simulink model "Xcvr_SSB_AM_2p5"  (Simulink 7.4)
settings: Solver=VariableStepDiscrete  SolverMode=SingleTasking  StartTime=0.0  StopTime=10  RelTol=1e-3
PreLoadFcn:
  | Fs=80e6;
  | 
  | phee=da_rom();
  | [phee_1,phee_2]=da_i2_rom();
  | 
  | Dcic=64;       % CIC decimation
  | Dfac=128;    % following DA filter decimation
  | N = 6;           %       (2^(N+1))=Dfac
  | Daudio=Dcic*Dfac;
  | Faudio=Fs/Daudio;
  | 
  | load info_filt_ssb_4
  | load Serial_Intfc_Stream_5
  | 
  | % AGC related
  | x=0.5:1/256:(1-1/256);
  | addr=(x-0.5)*256;
  | y=1./x;
undefined symbols (not defined in the file): Serial_Interface, ssb_coef, xlipgetpartsetting
libraries: xbsIndex_r4 x1305, dspsrcs4 x5, simulink x2, dspsigops x2, dspsnks4 x1
(part 2 of 11)

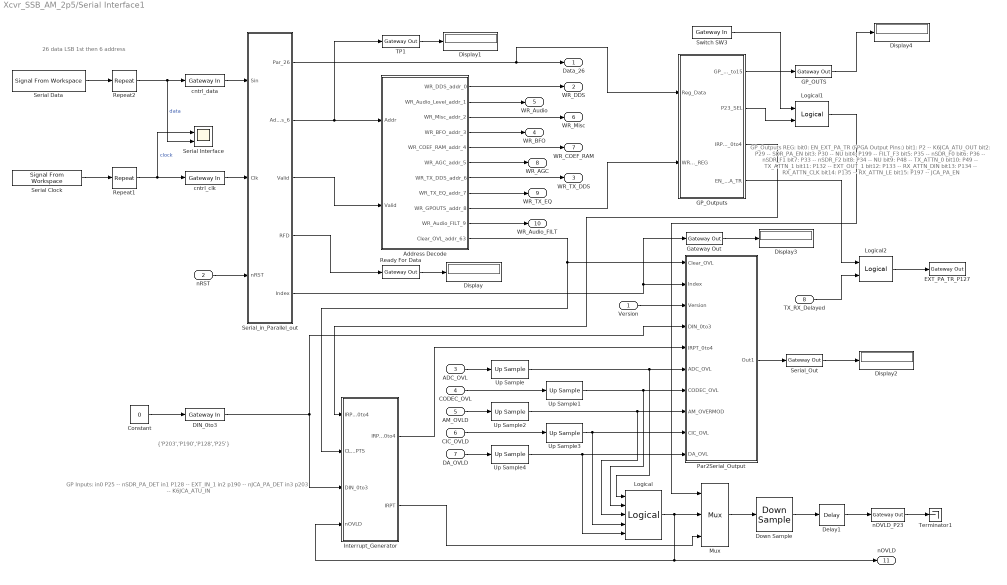
== system Xcvr_SSB_AM_2p5/Serial Interface1 ==
  note: 26 data  LSB 1st
      | then 6 address
  note: {'P203','P190','P128','P25'}
  note: GP Inputs:
      | in0  P25 -- nSDR_PA_DET
      | in1  P128 -- EXT_IN_1
      | in2  p190 -- nJCA_PA_DET
      | in3  p203 -- K6JCA_ATU_IN
  note: GP_Outputs REG:
      |
      | bit0: EN_EXT_PA_TR
      |
      | (FPGA Output Pins:)
      | bit1: P2 -- K6JCA_ATU_OUT
      | bit2: P29 -- SDR_PA_EN
      | bit3: P30 -- NU
      | bit4: P199 -- FILT_F3
      | bit5: P35 --  nSDR_F0
      | bit6: P36 -- nSDR_F1
      | bit7: P33 -- nSDR_F2
      | bit8: P34 -- NU
      |
      | bit9: P48 -- TX_ATTN_0
      | bit10: P49 -- TX_ATTN_1
      | bit11: P132 -- EXT_OUT_1
      | bit12: P133 -- RX_ATTN_DIN
      | bit13: P134 -- RX_ATTN_CLK
      | bit14: P135 -- RX_ATTN_LE
      | bit15: P197 -- JCA_PA_EN
  Version : Inport  OutDataType=fixdt(1, 16)  OutScaling=2^0
  nRST : Inport  Port=2  OutDataType=fixdt(1, 16)  OutScaling=2^0
  ADC_OVL : Inport  Port=3  OutDataType=fixdt(1, 16)  OutScaling=2^0
  CODEC_OVL : Inport  Port=4  OutDataType=fixdt(1, 16)  OutScaling=2^0
  AM_OVLD : Inport  Port=5  OutDataType=fixdt(1, 16)  OutScaling=2^0
  CIC_OVLD : Inport  Port=6  OutDataType=fixdt(1, 16)  OutScaling=2^0
  DA_OVLD : Inport  Port=7  OutDataType=fixdt(1, 16)  OutScaling=2^0
  TX_RX_Delayed : Inport  Port=8  OutDataType=fixdt(1, 16)  OutScaling=2^0
  Address Decode : Subsystem
  Constant : Constant  Value=0  OutDataType=fixdt(1, 16)  OutScaling=2^0  SampleTime=8/Fs
  DIN_0to3 : xbsIndex_r4/Gateway In  arith_type=Unsigned  n_bits=4  bin_pt=0  quantization="Round  (unbiased: +/- Inf)"  overflow=Wrap  period=8/Fs  dbl_ovrd=off  timing_constraint=None  locs_specified=on  LOCs={'P203','P190','P128','P25'}  hdl_port=on  block_type=gatewayin
      settings: infoedit="Gateway in block.  Converts inputs of type Simulink integer, double and fixed point to  Xilinx fixed point type.<br><br>Hardware notes:  In hardware these blocks become top level input ports."  block_version=9.2.00
  Delay1 : xbsIndex_r4/Delay  en=off  latency=1  dbl_ovrd=off  reg_retiming=off  block_type=delay
      settings: block_version=12.1
  Display{,1..4} (5 alike) : Display
  Down Sample : xbsIndex_r4/Down Sample  sample_ratio=1024  sample_phase="Last Value of Frame  (most efficient)"  en=off  latency=1  dbl_ovrd=off  block_type=dsamp
      settings: block_version=12.1
  EXT_PA_TR_P127 : xbsIndex_r4/Gateway Out  hdl_port=on  timing_constraint=None  locs_specified=on  LOCs={'P127'}  block_type=gatewayout
      settings: infoedit="Gateway out block.  Converts Xilinx fixed point inputs into ouputs of type Simulink integer, double, or fixed point.<br><br>Hardware notes:  In hardware these blocks become top level output ports or are discarded, depending on how they are configured."  block_version=12.1
  GP_OUTS : xbsIndex_r4/Gateway Out  hdl_port=on  timing_constraint=None  locs_specified=on  LOCs={'P197','P135','P134','P133','P132','P49','P48','P34','P33','P36','P35','P199','P30','P29','P2'}  block_type=gatewayout
      settings: infoedit="Gateway out block.  Converts Xilinx fixed point inputs into ouputs of type Simulink integer, double, or fixed point.<br><br>Hardware notes:  In hardware these blocks become top level output ports or are discarded, depending on how they are configured."  block_version=12.1
  GP_Outputs : Subsystem
  Gateway Out : xbsIndex_r4/Gateway Out  hdl_port=off  timing_constraint=None  locs_specified=off  LOCs={}  block_type=gatewayout
      settings: infoedit="Gateway out block.  Converts Xilinx fixed point inputs into ouputs of type Simulink integer, double, or fixed point.<br><br>Hardware notes:  In hardware these blocks become top level output ports or are discarded, depending on how they are configured."  block_version=12.1
  Interrupt_Generator : Subsystem
  Logical : xbsIndex_r4/Logical  logical_function=NOR  inputs=5  en=off  latency=0  precision=Full  arith_type=Unsigned  n_bits=16  bin_pt=0  align_bp=on  dbl_ovrd=off  block_type=logical
      settings: block_version=12.1
  Logical1 : xbsIndex_r4/Logical  logical_function=OR  inputs=2  en=off  latency=0  precision=Full  arith_type=Unsigned  n_bits=16  bin_pt=0  align_bp=on  dbl_ovrd=off  block_type=logical
      settings: block_version=12.1
  Logical2 : xbsIndex_r4/Logical  logical_function=AND  inputs=2  en=off  latency=0  precision=Full  arith_type=Unsigned  n_bits=16  bin_pt=0  align_bp=on  dbl_ovrd=off  block_type=logical
      settings: block_version=12.1
  Mux : xbsIndex_r4/Mux  inputs=2  en=off  latency=0  precision=Full  arith_type=Unsigned  n_bits=16  bin_pt=14  quantization=Truncate  overflow=Wrap  dbl_ovrd=off  block_type=mux
      settings: block_version=12.1
  Par2Serial_Output : Subsystem
  Ready For Data : xbsIndex_r4/Gateway Out  hdl_port=on  timing_constraint=None  locs_specified=on  LOCs={'P18'}  block_type=gatewayout
      settings: infoedit="Gateway out block.  Converts Xilinx fixed point inputs into ouputs of type Simulink integer, double, or fixed point.<br><br>Hardware notes:  In hardware these blocks become top level output ports or are discarded, depending on how they are configured."  block_version=12.1
  Repeat1 : dspsigops/Repeat  N=3*6  ic=0  mode=Maintain input frame size
  Repeat2 : dspsigops/Repeat  N=3*6  ic=0  mode=Maintain input frame size
  "Serial Clock  " : dspsrcs4/Signal From Workspace  SystemSampleTime=-1  X=Serial_Interface(1,:)  Ts=3*48/Fs  nsamps=1  OutputAfterFinalValue=Holding final value  ignoreOrWarnInputAndFrameLengths=off
  Serial Data : dspsrcs4/Signal From Workspace  SystemSampleTime=-1  X=Serial_Interface(2,:)  Ts=3*48/Fs  nsamps=1  OutputAfterFinalValue=Holding final value  ignoreOrWarnInputAndFrameLengths=off
  Serial Interface : Scope  NumInputPorts=2
      settings: YMin=-5~-5  YMax=5~5  SaveName=ScopeData3
  Serial_Out : xbsIndex_r4/Gateway Out  hdl_port=on  timing_constraint=None  locs_specified=on  LOCs={'P19'}  block_type=gatewayout
      settings: infoedit="Gateway out block.  Converts Xilinx fixed point inputs into ouputs of type Simulink integer, double, or fixed point.<br><br>Hardware notes:  In hardware these blocks become top level output ports or are discarded, depending on how they are configured."  block_version=12.1
  Serial_in_Parallel_out : Subsystem
  Switch SW3 : xbsIndex_r4/Gateway In  arith_type=Boolean  n_bits=1  bin_pt=0  quantization="Round  (unbiased: +/- Inf)"  overflow=Saturate  period=1/Faudio  dbl_ovrd=off  timing_constraint=None  locs_specified=on  LOCs={'P90'}  hdl_port=on  block_type=gatewayin
      settings: infoedit="Gateway in block.  Converts inputs of type Simulink integer, double and fixed point to  Xilinx fixed point type.<br><br>Hardware notes:  In hardware these blocks become top level input ports."  block_version=9.2.00
  TP1 : xbsIndex_r4/Gateway Out  hdl_port=off  timing_constraint=None  locs_specified=off  LOCs={'P11'}  block_type=gatewayout
      settings: infoedit="Gateway out block.  Converts Xilinx fixed point inputs into ouputs of type Simulink integer, double, or fixed point.<br><br>Hardware notes:  In hardware these blocks become top level output ports or are discarded, depending on how they are configured."  block_version=12.1
  Terminator1 : Terminator
  Up Sample : xbsIndex_r4/Up Sample  sample_ratio=8  copy_samples=on  en=off  latency=0  dbl_ovrd=off  block_type=usamp
      settings: block_version=12.1
  Up Sample1 : xbsIndex_r4/Up Sample  sample_ratio=1024  copy_samples=on  en=off  latency=0  dbl_ovrd=off  block_type=usamp
      settings: block_version=12.1
  Up Sample2 : xbsIndex_r4/Up Sample  sample_ratio=1024  copy_samples=on  en=off  latency=0  dbl_ovrd=off  block_type=usamp
      settings: block_version=12.1
  Up Sample3 : xbsIndex_r4/Up Sample  sample_ratio=8  copy_samples=on  en=off  latency=0  dbl_ovrd=off  block_type=usamp
      settings: block_version=12.1
  Up Sample4 : xbsIndex_r4/Up Sample  sample_ratio=8  copy_samples=on  en=off  latency=0  dbl_ovrd=off  block_type=usamp
      settings: block_version=12.1
  cntrl_clk : xbsIndex_r4/Gateway In  arith_type=Boolean  n_bits=16  bin_pt=14  quantization="Round  (unbiased: +/- Inf)"  overflow=Saturate  period=8/Fs  dbl_ovrd=off  timing_constraint=None  locs_specified=on  LOCs={'P16'}  hdl_port=on  block_type=gatewayin
      settings: infoedit="Gateway in block.  Converts inputs of type Simulink integer, double and fixed point to  Xilinx fixed point type.<br><br>Hardware notes:  In hardware these blocks become top level input ports."  block_version=9.2.00
  cntrl_data : xbsIndex_r4/Gateway In  arith_type=Boolean  n_bits=16  bin_pt=14  quantization="Round  (unbiased: +/- Inf)"  overflow=Saturate  period=8/Fs  dbl_ovrd=off  timing_constraint=None  locs_specified=on  LOCs={'P15'}  hdl_port=on  block_type=gatewayin
      settings: infoedit="Gateway in block.  Converts inputs of type Simulink integer, double and fixed point to  Xilinx fixed point type.<br><br>Hardware notes:  In hardware these blocks become top level input ports."  block_version=9.2.00
  nOVLD_P23 : xbsIndex_r4/Gateway Out  hdl_port=on  timing_constraint=None  locs_specified=on  LOCs={'P23'}  block_type=gatewayout
      settings: infoedit="Gateway out block.  Converts Xilinx fixed point inputs into ouputs of type Simulink integer, double, or fixed point.<br><br>Hardware notes:  In hardware these blocks become top level output ports or are discarded, depending on how they are configured."  block_version=9.2.00
  Data_26 : Outport
  WR_DDS : Outport  Port=2
  WR_TX_DDS : Outport  Port=3
  WR_BFO : Outport  Port=4
  WR_Audio : Outport  Port=5
  WR_Misc : Outport  Port=6
  WR_COEF_RAM : Outport  Port=7
  WR_AGC : Outport  Port=8
  WR_TX_EQ : Outport  Port=9
  WR_Audio_FILT : Outport  Port=10
  nOVLD : Outport  Port=11
  wires:
  cntrl_data/1 -> Serial_in_Parallel_out/1(Sin)
  cntrl_clk/1 -> Serial_in_Parallel_out/2(Clk)
  Serial_in_Parallel_out/2(Address_6) -> Address Decode/1(Addr), TP1/1
  Serial_in_Parallel_out/3(Valid) -> Address Decode/2(Valid)
  Address Decode/2(WR_Audio_Level_addr_1) -> WR_Audio/1
  Serial_in_Parallel_out/1(Par_26) -> Data_26/1, GP_Outputs/1(Reg_Data)
  Address Decode/1(WR_DDS_addr_0) -> WR_DDS/1
  Address Decode/4(WR_BFO_addr_3) -> WR_BFO/1
  Address Decode/3(WR_Misc_addr_2) -> WR_Misc/1
  Address Decode/5(WR_COEF_RAM_addr_4) -> WR_COEF_RAM/1
  Repeat2/1 -> Serial Interface/2, cntrl_data/1  "data"
  Serial Data/1 -> Repeat2/1
  "Serial Clock  "/1 -> Repeat1/1
  Repeat1/1 -> Serial Interface/1, cntrl_clk/1  "clock"
  Ready For Data/1 -> Display/1
  Serial_in_Parallel_out/4(RFD) -> Ready For Data/1
  TP1/1 -> Display1/1
  Serial_in_Parallel_out/5(Index) -> Par2Serial_Output/2(Index), Gateway Out/1
  DIN_0to3/1 -> Par2Serial_Output/4(DIN_0to3), Interrupt_Generator/3(DIN_0to3)
  Version/1 -> Par2Serial_Output/3(Version)
  Par2Serial_Output/1(Out1) -> Serial_Out/1
  Serial_Out/1 -> Display2/1
  Constant/1 -> DIN_0to3/1
  ADC_OVL/1 -> Up Sample/1
  CODEC_OVL/1 -> Up Sample1/1
  Gateway Out/1 -> Display3/1
  Up Sample/1 -> Par2Serial_Output/6(ADC_OVL), Logical/1
  Up Sample1/1 -> Par2Serial_Output/7(CODEC_OVL), Logical/2
  Up Sample2/1 -> Par2Serial_Output/8(AM_OVERMOD), Logical/3
  AM_OVLD/1 -> Up Sample2/1
  Up Sample3/1 -> Par2Serial_Output/9(CIC_OVL), Logical/4
  CIC_OVLD/1 -> Up Sample3/1
  Up Sample4/1 -> Par2Serial_Output/10(DA_OVL), Logical/5
  DA_OVLD/1 -> Up Sample4/1
  Address Decode/6(WR_AGC_addr_5) -> WR_AGC/1
  Address Decode/7(WR_TX_DDS_addr_6) -> WR_TX_DDS/1
  nRST/1 -> Serial_in_Parallel_out/3(nRST)
  nOVLD_P23/1 -> Terminator1/1
  Delay1/1 -> nOVLD_P23/1
  Logical/1 -> Mux/2, Interrupt_Generator/4(nOVLD), nOVLD/1
  Interrupt_Generator/2(IRPT) -> Mux/3
  Interrupt_Generator/1(IRPT_0to4) -> Par2Serial_Output/5(IRPT_0to4)
  GP_Outputs/2(P23_SEL) -> Logical1/2
  Switch SW3/1 -> Logical1/1
  Logical1/1 -> Mux/1
  GP_Outputs/1(GP_OUT_BIT_1_to15) -> GP_OUTS/1
  GP_OUTS/1 -> Display4/1
  Mux/1 -> Down Sample/1
  Down Sample/1 -> Delay1/1
  GP_Outputs/3(IRPT_EN_0to4) -> Interrupt_Generator/1(IRPT_EN_0to4)
  Address Decode/8(WR_TX_EQ_addr_7) -> WR_TX_EQ/1
  Address Decode/9(WR_GPOUTS_addr_8) -> GP_Outputs/2(WR_GP_REG)
  Address Decode/11(Clear_OVL_addr_63) -> Par2Serial_Output/1(Clear_OVL), Interrupt_Generator/2(CLR_IRPTS)
  Address Decode/10(WR_Audio_FILT_9) -> WR_Audio_FILT/1
  Logical2/1 -> EXT_PA_TR_P127/1
  GP_Outputs/4(EN_EXT_PA_TR) -> Logical2/1
  TX_RX_Delayed/1 -> Logical2/2

== system Xcvr_SSB_AM_2p5/TX Filters I=8192 ==
  Real_In : Inport
  Imag_In : Inport  Port=2
  " Sample Rate" : Display
  " Sample Rate1" : Display
  "CIC Compiler 2.0 " : xbsIndex_r4/CIC Compiler 2.0   filter_type=Interpolation  number_of_stages=5  differential_delay=1  number_of_channels=1  sample_rate_changes=Fixed  fixed_or_initial_rate=64  minimum_rate=4  maximum_rate=4  ratespecification=Hardware_Oversampling_Rate  sampleperiod=4  hardwareoversamplingrate=1  quantization=Truncation  output_data_width=16  use_xtreme_dsp_slice=on  use_streaming_interface=on  sclr=off  ce=off  gui_behaviour=Sysgen  input_data_width=18  ip_name=CIC Compiler  ip_version=2.0  dsptool_ready=true  wrapper_available=true  port_translation_map={ 'ce' => 'en', 'sclr' => 'rst' }  ipcore_xco_need_fpga_part=true  ipcore_fpga_part=xlipgetpartsetting(gcb, {'virtex4', 'xc4vsx35', '-10', 'ff668'})  ipcore_verbose=false  block_type=cic_compiler_v2_0
      settings: block_version=12.1
  CIC Compiler 2.0 1 : xbsIndex_r4/CIC Compiler 2.0   filter_type=Interpolation  number_of_stages=5  differential_delay=1  number_of_channels=1  sample_rate_changes=Fixed  fixed_or_initial_rate=64  minimum_rate=4  maximum_rate=4  ratespecification=Hardware_Oversampling_Rate  sampleperiod=4  hardwareoversamplingrate=1  quantization=Truncation  output_data_width=16  use_xtreme_dsp_slice=on  use_streaming_interface=on  sclr=off  ce=off  gui_behaviour=Sysgen  input_data_width=18  ip_name=CIC Compiler  ip_version=2.0  dsptool_ready=true  wrapper_available=true  port_translation_map={ 'ce' => 'en', 'sclr' => 'rst' }  ipcore_xco_need_fpga_part=true  ipcore_fpga_part=xlipgetpartsetting(gcb, {'virtex4', 'xc4vsx35', '-10', 'ff668'})  ipcore_verbose=false  block_type=cic_compiler_v2_0
      settings: block_version=12.1
  Commutator : Subsystem
  Control : Subsystem
  Convert : xbsIndex_r4/Convert  arith_type="Signed  (2's comp)"  n_bits=16  bin_pt=15  quantization=Truncate  overflow=Wrap  en=off  latency=0  dbl_ovrd=off  pipeline=off  block_type=convert
      settings: block_version=12.2
  Convert1 : xbsIndex_r4/Convert  arith_type="Signed  (2's comp)"  n_bits=16  bin_pt=15  quantization=Truncate  overflow=Wrap  en=off  latency=0  dbl_ovrd=off  pipeline=off  block_type=convert
      settings: block_version=12.2
  Delay1 : xbsIndex_r4/Delay  en=off  latency=1  dbl_ovrd=off  reg_retiming=off  block_type=delay
      settings: block_version=9.2.00
  Delay2 : xbsIndex_r4/Delay  en=off  latency=1  dbl_ovrd=off  reg_retiming=off  block_type=delay
      settings: block_version=9.2.00
  Fs_probe_1 : Subsystem
  Fs_probe_2 : Subsystem
  IO_Control : Subsystem
  Ifac=2^(N+1) : xbsIndex_r4/Constant  arith_type=Unsigned  const=N  n_bits=3  bin_pt=0  explicit_period=on  period=1/Fs  equ=P=C  opselect=C  inp2=PCIN>>17  opr=+  inp1=P  carry=CIN  dbl_ovrd=off  block_type=constant
      settings: block_version=9.2.00
  Interp_Core : Subsystem
  Register : xbsIndex_r4/Register  init=0  rst=off  en=on  dbl_ovrd=off  block_type=register
      settings: block_version=12.1
  Register1 : xbsIndex_r4/Register  init=0  rst=off  en=on  dbl_ovrd=off  block_type=register
      settings: block_version=12.1
  Reinterpret1 : xbsIndex_r4/Reinterpret  force_arith_type=on  arith_type="Signed  (2's comp)"  force_bin_pt=on  bin_pt=15  block_type=reinterpret
      settings: infoedit="Changes signal type without altering the binary representation.   You can changed the signal between signed and unsigned, and relocate the binary point.<br><br>Hardware notes: In hardware this block costs nothing.<br><br>Example:  Suppose the input is 6 bits wide, signed, with 2 fractional bits, and the output is forced to unsigned with 0 fractional bits.  Then an input of -2.0 (1110.00 in binary 2's complement) becomes an output of 56 (111000 in binary)."  block_version=12.1
  Reinterpret2 : xbsIndex_r4/Reinterpret  force_arith_type=on  arith_type="Signed  (2's comp)"  force_bin_pt=on  bin_pt=15  block_type=reinterpret
      settings: infoedit="Changes signal type without altering the binary representation.   You can changed the signal between signed and unsigned, and relocate the binary point.<br><br>Hardware notes: In hardware this block costs nothing.<br><br>Example:  Suppose the input is 6 bits wide, signed, with 2 fractional bits, and the output is forced to unsigned with 0 fractional bits.  Then an input of -2.0 (1110.00 in binary 2's complement) becomes an output of 56 (111000 in binary)."  block_version=12.1
  TP : xbsIndex_r4/Gateway Out  hdl_port=off  timing_constraint=None  locs_specified=off  LOCs={ 'b15','c15','c16','d14','b4','e13','k1','g1'}  block_type=gatewayout
      settings: infoedit="Gateway out block.  Converts Xilinx fixed point inputs into ouputs of type Simulink integer, double, or fixed point.<br><br>Hardware notes:  In hardware these blocks become top level output ports or are discarded, depending on how they are configured."  block_version=9.2.00
  TP1 : xbsIndex_r4/Gateway Out  hdl_port=off  timing_constraint=None  locs_specified=off  LOCs={ 'b15','c15','c16','d14','b4','e13','k1','g1'}  block_type=gatewayout
      settings: infoedit="Gateway out block.  Converts Xilinx fixed point inputs into ouputs of type Simulink integer, double, or fixed point.<br><br>Hardware notes:  In hardware these blocks become top level output ports or are discarded, depending on how they are configured."  block_version=9.2.00
  Terminator : Terminator
  Terminator2 : Terminator
  Tx_Iout : Outport
  Tx_Qout : Outport  Port=2
  wires:
  Delay1/1 -> IO_Control/4(Imag_In)
  Delay2/1 -> IO_Control/3(Real_In)
  Interp_Core/1(Yn1_out) -> IO_Control/1(Yn1), Commutator/1(Yn1)
  Interp_Core/2(Yn2_out) -> IO_Control/2(Yn2), Commutator/2(Yn2)
  IO_Control/1(Xout) -> Interp_Core/1(Xin)
  Control/3(AB_Write) -> IO_Control/7(Write)
  Control/6(Start) -> Interp_Core/2(Start)
  Control/7(SR_Addr) -> Interp_Core/3(SR_Addr)
  Control/5(AB_Sel) -> IO_Control/9(AB_Sel)
  Control/1(AB_Addr) -> IO_Control/5(AB_Addr)
  Interp_Core/3(Valid) -> Control/1(Valid)
  Control/4(Real_Imag) -> IO_Control/8(Real_Imag)
  Control/2(In_Sel) -> IO_Control/6(In_sel)
  Commutator/1(Real) -> "CIC Compiler 2.0 "/1
  Commutator/2(Imag) -> CIC Compiler 2.0 1/1, TP/1
  Real_In/1 -> TP1/1, Convert/1
  Ifac=2^(N+1)/1 -> Control/2(Ifac)
  "CIC Compiler 2.0 "/1 -> Reinterpret1/1
  CIC Compiler 2.0 1/1 -> Reinterpret2/1
  "CIC Compiler 2.0 "/2 -> Terminator/1
  "CIC Compiler 2.0 "/3 -> Register/2
  CIC Compiler 2.0 1/2 -> Terminator2/1
  CIC Compiler 2.0 1/3 -> Register1/2
  Reinterpret1/1 -> Register/1
  Register/1 -> Tx_Iout/1
  Register1/1 -> Tx_Qout/1
  Reinterpret2/1 -> Register1/1
  Fs_probe_1/1(Out1) -> " Sample Rate"/1
  TP/1 -> Fs_probe_1/1(In1)
  Fs_probe_2/1(Out1) -> " Sample Rate1"/1
  TP1/1 -> Fs_probe_2/1(In1)
  Convert/1 -> Delay2/1
  Convert1/1 -> Delay1/1
  Imag_In/1 -> Convert1/1

== system Xcvr_SSB_AM_2p5/Up/Down LO and Mixers ==
  note: ADC or DAC Potential Overload
  ADC In : Inport  OutDataType=fixdt(1, 16)  OutScaling=2^0
  I_Tx : Inport  Port=2  OutDataType=fixdt(1, 16)  OutScaling=2^0
  Q_Tx1 : Inport  Port=3  OutDataType=fixdt(1, 16)  OutScaling=2^0
  LO_DDS_Data : Inport  Port=4  OutDataType=fixdt(1, 16)  OutScaling=2^0
  RXLO_DDS_Write : Inport  Port=5  OutDataType=fixdt(1, 16)  OutScaling=2^0
  TXLO_DDS_Write : Inport  Port=6  OutDataType=fixdt(1, 16)  OutScaling=2^0
  Tx_Rx_Delayed : Inport  Port=7
  Assert : xbsIndex_r4/Assert  assert_type=off  type_source=Explicitly  arith_type="Signed  (2's comp)"  n_bits=16  bin_pt=14  assert_rate=on  rate_source=Explicitly  period=1/Fs  output_port=on  block_type=assert
      settings: block_version=12.1
  CMult : xbsIndex_r4/CMult  const=2  const_n_bits=2  const_bin_pt=0  en=off  latency=1  precision=User Defined  arith_type="Signed  (2's comp)"  n_bits=14  bin_pt=13  quantization="Round  (unbiased: +/- Inf)"  overflow=Saturate  dbl_ovrd=off  use_behavioral_HDL=off  mem_type=Distributed RAM  pipeline=off  block_type=cmult
      settings: block_version=12.1
  DDS_LO : Subsystem
  Delay allow T/R  Relay time. : Subsystem
  Inverter : xbsIndex_r4/Inverter  en=off  latency=0  dbl_ovrd=off  block_type=inv
      settings: block_version=12.1
  Mult : xbsIndex_r4/Mult  precision=User Defined  arith_type="Signed  (2's comp)"  n_bits=16  bin_pt=15  quantization="Round  (unbiased: +/- Inf)"  overflow=Wrap  en=on  latency=3  dbl_ovrd=off  use_behavioral_HDL=off  opt=Speed  use_embedded=on  optimum_pipeline=off  pipeline=on  use_rpm=on  placement_style=Triangular  block_type=mult
      settings: block_version=9.2.00
  Mult1 : xbsIndex_r4/Mult  precision=User Defined  arith_type="Signed  (2's comp)"  n_bits=16  bin_pt=15  quantization="Round  (unbiased: +/- Inf)"  overflow=Wrap  en=on  latency=3  dbl_ovrd=off  use_behavioral_HDL=off  opt=Speed  use_embedded=on  optimum_pipeline=off  pipeline=on  use_rpm=on  placement_style=Triangular  block_type=mult
      settings: block_version=9.2.00
  Mux : xbsIndex_r4/Mux  inputs=2  en=off  latency=1  precision=Full  arith_type=Unsigned  n_bits=16  bin_pt=14  quantization=Truncate  overflow=Wrap  dbl_ovrd=off  block_type=mux
      settings: block_version=12.1
  Mux1 : xbsIndex_r4/Mux  inputs=2  en=off  latency=1  precision=Full  arith_type=Unsigned  n_bits=16  bin_pt=14  quantization=Truncate  overflow=Wrap  dbl_ovrd=off  block_type=mux
      settings: block_version=12.1
  Mux2 : xbsIndex_r4/Mux  inputs=2  en=off  latency=1  precision=Full  arith_type=Unsigned  n_bits=16  bin_pt=14  quantization=Truncate  overflow=Wrap  dbl_ovrd=off  block_type=mux
      settings: block_version=12.1
  OverLoad_Det : Subsystem
  RX_I : xbsIndex_r4/Register  init=0  rst=on  en=off  dbl_ovrd=off  block_type=register
      settings: block_version=9.2.00
  RX_Q : xbsIndex_r4/Register  init=0  rst=on  en=off  dbl_ovrd=off  block_type=register
      settings: block_version=9.2.00
  Register : xbsIndex_r4/Register  init=0  rst=on  en=off  dbl_ovrd=off  block_type=register
      settings: block_version=9.2.00
  Register1 : xbsIndex_r4/Register  init=0  rst=on  en=off  dbl_ovrd=off  block_type=register
      settings: block_version=9.2.00
  TX_Add : xbsIndex_r4/AddSub  mode=Addition  use_carryin=off  use_carryout=off  en=off  latency=0  precision=User Defined  arith_type="Signed  (2's comp)"  n_bits=16  bin_pt=15  quantization="Round  (unbiased: +/- Inf)"  overflow=Saturate  dbl_ovrd=off  use_behavioral_HDL=off  hw_selection=Fabric  pipelined=off  block_type=addsub
      settings: block_version=12.1
  I_Rx : Outport  OutDataType=fixdt(1, 16)  OutScaling=2^0
  Q_Rx1 : Outport  Port=2  OutDataType=fixdt(1, 16)  OutScaling=2^0
  Tx_Out : Outport  Port=3  OutDataType=fixdt(1, 16)  OutScaling=2^0
  ADC_OVL : Outport  Port=4
  wires:
  DDS_LO/2(Out2) -> Mult1/2
  DDS_LO/3(Out3) -> Mult/2
  DDS_LO/1(Out1) -> Mult1/3, Mult/3
  ADC In/1 -> Register/1
  Mux/1 -> Mult/1
  Mux1/1 -> Mult1/1
  Register/1 -> Mux/2, Mux1/2, Mux2/2
  I_Tx/1 -> Mux/3
  Q_Tx1/1 -> Mux1/3
  Mult1/1 -> TX_Add/2, RX_Q/1
  Mult/1 -> TX_Add/1, RX_I/1
  TX_Add/1 -> CMult/1
  Register1/1 -> Tx_Out/1
  Tx_Rx_Delayed/1 -> Mux1/1, Mux/1, Mux2/1, Inverter/1, RX_I/2, RX_Q/2, DDS_LO/1(Tx_Rx_Delayed), Delay allow T/R  Relay time./1(Tx_Rx_Delayed)
  OverLoad_Det/1(Out1) -> ADC_OVL/1
  Assert/1 -> Register1/1
  Inverter/1 -> Register1/2
  CMult/1 -> Assert/1, Mux2/3
  RX_I/1 -> I_Rx/1
  RX_Q/1 -> Q_Rx1/1
  LO_DDS_Data/1 -> DDS_LO/4(Data)
  RXLO_DDS_Write/1 -> DDS_LO/2(RX_Write)
  TXLO_DDS_Write/1 -> DDS_LO/3(TX_Write)
  Delay allow T/R  Relay time./1(ADC_OFF) -> Register/2
  Mux2/1 -> OverLoad_Det/1(In1)

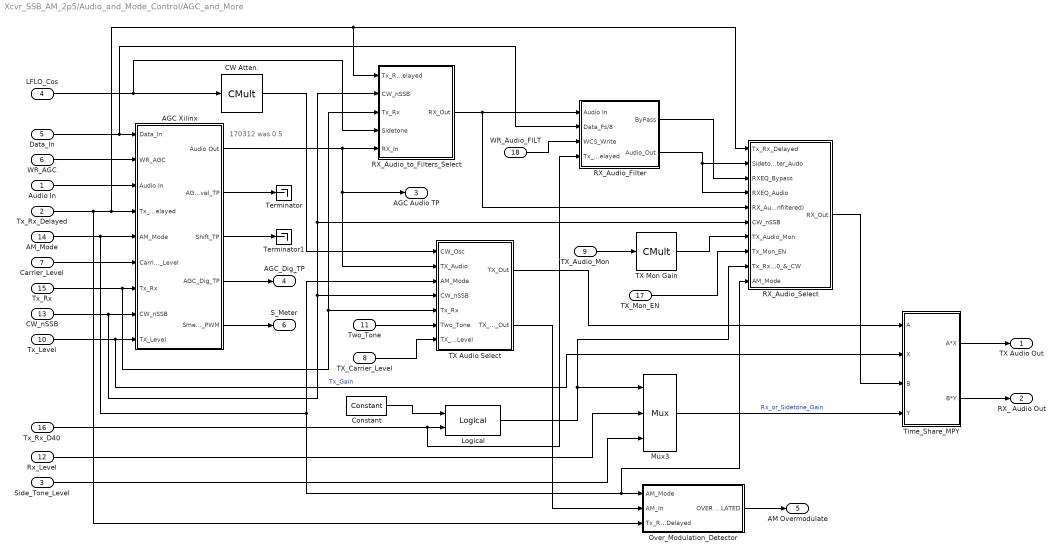
== system Xcvr_SSB_AM_2p5/Audio_and_Mode_Control/AGC_and_More ==
  note: 170312 was 0.5
  Audio In : Inport
  Tx_Rx_Delayed : Inport  Port=2
  Side_Tone_Level : Inport  Port=3
  LFLO_Cos : Inport  Port=4
  Data_In : Inport  Port=5
  WR_AGC : Inport  Port=6
  Carrier_Level : Inport  Port=7
  TX_Carrier_Level : Inport  Port=8
  TX_Audio_Mon : Inport  Port=9
  Tx_Level : Inport  Port=10
  Two_Tone : Inport  Port=11
  Rx_Level : Inport  Port=12
  CW_nSSB : Inport  Port=13
  AM_Mode : Inport  Port=14
  Tx_Rx : Inport  Port=15
  Tx_Rx_D40 : Inport  Port=16
  TX_Mon_EN : Inport  Port=17
  WR_Audio_FILT : Inport  Port=18
  AGC Xilinx : Subsystem
  CW Atten. : xbsIndex_r4/CMult  const=1.0  const_n_bits=3  const_bin_pt=2  en=off  latency=0  precision=User Defined  arith_type="Signed  (2's comp)"  n_bits=16  bin_pt=15  quantization=Truncate  overflow=Saturate  dbl_ovrd=off  use_behavioral_HDL=off  mem_type=Distributed RAM  pipeline=off  use_rpm=off  placement_style=Rectangular Shape  block_type=cmult
      settings: block_version=9.2.00
  Constant : xbsIndex_r4/Constant  arith_type=Boolean  const=1  n_bits=16  bin_pt=14  explicit_period=off  period=1  equ=P=C  opselect=C  inp2=PCIN>>17  opr=+  inp1=P  carry=CIN  dbl_ovrd=off  block_type=constant
      settings: block_version=12.2
  Logical : xbsIndex_r4/Logical  logical_function=AND  inputs=2  en=off  latency=0  precision=Full  arith_type=Unsigned  n_bits=16  bin_pt=0  align_bp=on  dbl_ovrd=off  block_type=logical
      settings: block_version=9.2.00
  Mux3 : xbsIndex_r4/Mux  inputs=2  en=off  latency=0  precision=Full  arith_type=Unsigned  n_bits=32  bin_pt=32  quantization="Round  (unbiased: +/- Inf)"  overflow=Wrap  dbl_ovrd=off  block_type=mux
      settings: block_version=9.2.00
  Over_Modulation_Detector : Subsystem
  RX_Audio_Filter : Subsystem
  RX_Audio_Select : Subsystem
  RX_Audio_to_Filters_Select : Subsystem
  TX Audio Select : Subsystem
  TX Mon Gain : xbsIndex_r4/CMult  const=2  const_n_bits=3  const_bin_pt=1  en=off  latency=0  precision=User Defined  arith_type="Signed  (2's comp)"  n_bits=16  bin_pt=15  quantization=Truncate  overflow=Saturate  dbl_ovrd=off  use_behavioral_HDL=off  mem_type=Distributed RAM  pipeline=off  use_rpm=off  placement_style=Rectangular Shape  block_type=cmult
      settings: block_version=9.2.00
  Terminator : Terminator
  Terminator1 : Terminator
  Time_Share_MPY : Subsystem
  TX Audio Out : Outport
  RX_ Audio Out : Outport  Port=2
  AGC Audio TP : Outport  Port=3
  AGC_Dig_TP : Outport  Port=4
  AM Overmodulate : Outport  Port=5
  S_Meter : Outport  Port=6
  wires:
  Rx_Level/1 -> Mux3/2
  Tx_Level/1 -> AGC Xilinx/9(TX_Level), Time_Share_MPY/2(X)  "Tx_Gain"
  LFLO_Cos/1 -> CW Atten./1, RX_Audio_to_Filters_Select/4(Sidetone)
  Logical/1 -> RX_Audio_Select/9(Tx_Rx_D40_&_CW), Mux3/1
  Mux3/1 -> Time_Share_MPY/4(Y)  "Rx_or_Sidetone_Gain"
  Audio In/1 -> AGC Xilinx/3(Audio In)
  Side_Tone_Level/1 -> Mux3/3
  Tx_Rx/1 -> TX Audio Select/5(Tx_Rx), RX_Audio_to_Filters_Select/3(Tx_Rx), AGC Xilinx/7(Tx_Rx)
  AGC Xilinx/2(AGC_Level_TP) -> Terminator/1
  AGC Xilinx/3(Shift_TP) -> Terminator1/1
  Time_Share_MPY/1(A*X) -> TX Audio Out/1
  Time_Share_MPY/2(B*Y) -> RX_ Audio Out/1
  AM_Mode/1 -> AGC Xilinx/5(AM_Mode), TX Audio Select/3(AM_Mode), Over_Modulation_Detector/1(AM_Mode), RX_Audio_Select/10(AM_Mode)
  Carrier_Level/1 -> AGC Xilinx/6(Carrier_Level)
  Tx_Rx_Delayed/1 -> AGC Xilinx/4(Tx_Rx_Delayed), RX_Audio_to_Filters_Select/1(Tx_Rx_Delayed), RX_Audio_Select/1(Tx_Rx_Delayed), Over_Modulation_Detector/3(Tx_Rx_Delayed)
  AGC Xilinx/1(Audio Out) -> AGC Audio TP/1, TX Audio Select/2(TX_Audio), RX_Audio_to_Filters_Select/5(RX_In)
  AGC Xilinx/4(AGC_Dig_TP) -> AGC_Dig_TP/1
  WR_AGC/1 -> AGC Xilinx/2(WR_AGC)
  Data_In/1 -> AGC Xilinx/1(Data_In), RX_Audio_Filter/2(Data_Fs/8)
  CW_nSSB/1 -> AGC Xilinx/8(CW_nSSB), TX Audio Select/4(CW_nSSB), RX_Audio_to_Filters_Select/2(CW_nSSB), RX_Audio_Select/6(CW_nSSB)
  Over_Modulation_Detector/1(OVER MODULATED) -> AM Overmodulate/1
  Tx_Rx_D40/1 -> Logical/2, RX_Audio_Filter/4(Tx_Rx_Delayed)
  RX_Audio_to_Filters_Select/1(RX_Out) -> RX_Audio_Select/5(RX_Audio_(unfiltered)), RX_Audio_Filter/1(Audio In)
  TX Audio Select/2(TX_AM_Out) -> Over_Modulation_Detector/2(AM_In)
  TX Audio Select/1(TX_Out) -> Time_Share_MPY/1(A)
  Two_Tone/1 -> TX Audio Select/6(Two_Tone)
  CW Atten./1 -> TX Audio Select/1(CW_Osc)
  TX_Carrier_Level/1 -> TX Audio Select/7(TX_Carrier_Level)
  RX_Audio_Select/1(RX_Out) -> Time_Share_MPY/3(B)
  TX_Mon_EN/1 -> RX_Audio_Select/8(Tx_Mon_EN)
  AGC Xilinx/5(Smeter_PWM) -> S_Meter/1
  RX_Audio_Filter/2(Audio_Out) -> RX_Audio_Select/4(RXEQ_Audio), RX_Audio_Select/2(Sidetone_Filter_Audo)
  RX_Audio_Filter/1(ByPass) -> RX_Audio_Select/3(RXEQ_Bypass)
  WR_Audio_FILT/1 -> RX_Audio_Filter/3(WCS_Write)
  TX Mon Gain/1 -> RX_Audio_Select/7(TX_Audio_Mon)
  TX_Audio_Mon/1 -> TX Mon Gain/1
  Constant/1 -> Logical/1

== system Xcvr_SSB_AM_2p5/Audio_and_Mode_Control/Audio_Processor ==
  Manual_Activate_EQ : Inport
  CODEC_ADC : Inport  Port=2
  TX_WCS_Write : Inport  Port=3
  Data : Inport  Port=4
  Tx_Rx_Delayed : Inport  Port=5
  CW_nSSB : Inport  Port=6
  Inverter1 : xbsIndex_r4/Inverter  en=off  latency=0  dbl_ovrd=off  block_type=inv
      settings: block_version=9.2.00
  Mux : xbsIndex_r4/Mux  inputs=2  en=off  latency=0  precision=Full  arith_type=Unsigned  n_bits=16  bin_pt=14  quantization=Truncate  overflow=Wrap  dbl_ovrd=off  block_type=mux
      settings: block_version=12.1
  Mux1 : xbsIndex_r4/Mux  inputs=2  en=off  latency=0  precision=User Defined  arith_type="Signed  (2's comp)"  n_bits=16  bin_pt=15  quantization=Truncate  overflow=Wrap  dbl_ovrd=off  block_type=mux
      settings: block_version=12.1
  OVL_Detect : Subsystem
  Serial_to_Parallel : Subsystem
  TX Equalizer : Subsystem
  Audio_Out : Outport
  CODEC_OVL : Outport  Port=2
  wires:
  Serial_to_Parallel/2(R_out) -> Mux/3, Mux1/3  "Line_In"
  TX Equalizer/2(Audio_Out) -> Mux/2
  Serial_to_Parallel/1(L_out) -> TX Equalizer/2(Audio In), Mux1/2  "Mic_In"
  Data/1 -> TX Equalizer/3(Data_Fs/8)
  Manual_Activate_EQ/1 -> TX Equalizer/1(Activate)
  CODEC_ADC/1 -> Serial_to_Parallel/1(Serial_in)
  Mux/1 -> Audio_Out/1, OVL_Detect/3(Audio_Out)
  TX_WCS_Write/1 -> TX Equalizer/4(WCS_Write)
  TX Equalizer/1(Line_Select) -> Mux/1, Mux1/1
  OVL_Detect/1(OVL_Out) -> CODEC_OVL/1
  Tx_Rx_Delayed/1 -> Inverter1/1
  Inverter1/1 -> OVL_Detect/1(Reset)
  Mux1/1 -> OVL_Detect/2(Aud_In)
  CW_nSSB/1 -> TX Equalizer/5(CW_nSSB)

== system Xcvr_SSB_AM_2p5/Audio_and_Mode_Control/Codec T_C ==
  note: For PCM3008:  Sysclk toggles at Fs/32=2.5MHz for Fs=80e6.  This is 256*Fs_audio.
      | Fs_Audio = Fs/8192=9,765.625Hz for Fs=80e6;
  In1 : Inport
  Concat : xbsIndex_r4/Concat  num_inputs=5  dbl_ovrd=off  block_type=concat
      settings: block_version=9.2.00
  Counter Fclk=512*Fs_Audio : xbsIndex_r4/Counter  cnt_type=Free Running  cnt_to=Inf  operation=Up  start_count=0  cnt_by_val=1  arith_type=Unsigned  n_bits=10  bin_pt=0  load_pin=off  rst=off  en=off  explicit_period=on  period=16/Fs  dbl_ovrd=off  use_behavioral_HDL=off  implementation=Fabric  use_rpm=off  block_type=counter
      settings: block_version=9.2.00
  Inverter : xbsIndex_r4/Inverter  en=off  latency=0  dbl_ovrd=off  block_type=inv
      settings: block_version=9.2.00
  Power Down Control : Subsystem
  bit 0 : xbsIndex_r4/Slice  nbits=1  boolean_output=on  mode=Lower Bit Location + Width  bit1=0  base1=LSB of Input  bit0=0  base0=LSB of Input  dbl_ovrd=off  block_type=slice
      settings: infoedit="Extracts a given range of bits from each input sample and presents it at the output.  The output type is ordinarily unsigned with binary point at zero, but can be Boolean when the slice is one bit wide.<P><P>Hardware notes: In hardware this block costs nothing."  block_version=9.2.00
  bit 3 : xbsIndex_r4/Slice  nbits=1  boolean_output=on  mode=Lower Bit Location + Width  bit1=0  base1=LSB of Input  bit0=3  base0=LSB of Input  dbl_ovrd=off  block_type=slice
      settings: block_version=9.2.00
  bit 8 : xbsIndex_r4/Slice  nbits=1  boolean_output=on  mode=Lower Bit Location + Width  bit1=0  base1=LSB of Input  bit0=8  base0=LSB of Input  dbl_ovrd=off  block_type=slice
      settings: block_version=9.2.00
  bit 9 : xbsIndex_r4/Slice  nbits=1  boolean_output=on  mode=Lower Bit Location + Width  bit1=0  base1=LSB of Input  bit0=9  base0=LSB of Input  dbl_ovrd=off  block_type=slice
      settings: block_version=9.2.00
  Out1 : Outport
  wires:
  bit 8/1 -> Inverter/1  "lrclk"
  bit 3/1 -> Concat/3  "bclk"
  Counter Fclk=512*Fs_Audio/1 -> bit 0/1, bit 8/1, bit 3/1, bit 9/1
  bit 0/1 -> Concat/1  "sysclk"
  Power Down Control/1(Out1) -> Concat/5  "pd_bar"
  Inverter/1 -> Concat/2
  Concat/1 -> Out1/1
  In1/1 -> Concat/4
  bit 9/1 -> Power Down Control/1(In1)

== system Xcvr_SSB_AM_2p5/Audio_and_Mode_Control/Parallel_to_Serial ==
  Lin : Inport
  Rin : Inport  Port=2
  Concat : xbsIndex_r4/Concat  num_inputs=2  dbl_ovrd=off  block_type=concat
      settings: block_version=9.2.00
  Convert : xbsIndex_r4/Convert  arith_type=Boolean  n_bits=16  bin_pt=14  quantization=Truncate  overflow=Wrap  en=off  latency=0  dbl_ovrd=off  pipeline=off  block_type=convert
      settings: block_version=9.2.00
  Parallel to Serial : xbsIndex_r4/Parallel to Serial  output_order=Most Significant Word First  arith_type=Unsigned  output_bits=1  bin_pt=0  en=off  latency=0  dbl_ovrd=off  block_type=p2s
      settings: infoedit=Each sample presented at the input becomes several samples presented serially at the output.  block_version=9.2.00
  Reinterpret : xbsIndex_r4/Reinterpret  force_arith_type=on  arith_type=Unsigned  force_bin_pt=on  bin_pt=0  block_type=reinterpret
      settings: infoedit="Changes signal type without altering the binary representation.   You can changed the signal between signed and unsigned, and relocate the binary point.<P><P>Hardware notes: In hardware this block costs nothing.<P><P>Example:  Suppose the input is 6 bits wide, signed, with 2 fractional bits, and the output is forced to unsigned with 0 fractional bits.  Then an input of -2.0 (1110.00 in binary 2's complement) becomes an output of 56 (111000 in binary)."  block_version=9.2.00
  Reinterpret1 : xbsIndex_r4/Reinterpret  force_arith_type=on  arith_type=Unsigned  force_bin_pt=on  bin_pt=0  block_type=reinterpret
      settings: infoedit="Changes signal type without altering the binary representation.   You can changed the signal between signed and unsigned, and relocate the binary point.<P><P>Hardware notes: In hardware this block costs nothing.<P><P>Example:  Suppose the input is 6 bits wide, signed, with 2 fractional bits, and the output is forced to unsigned with 0 fractional bits.  Then an input of -2.0 (1110.00 in binary 2's complement) becomes an output of 56 (111000 in binary)."  block_version=9.2.00
  Serial_Out : Outport
  wires:
  Rin/1 -> Reinterpret1/1
  Parallel to Serial/1 -> Convert/1
  Concat/1 -> Parallel to Serial/1
  Lin/1 -> Reinterpret/1
  Reinterpret/1 -> Concat/1
  Reinterpret1/1 -> Concat/2
  Convert/1 -> Serial_Out/1

== system Xcvr_SSB_AM_2p5/Audio_and_Mode_Control/Reg_A ==
  note: Fs/8192
  note: Bits 10...19 Tx audio gain
  note: Bits 0..9 for RX audio gain control
  note: Bits 0..9 for RX audio gain control
      | Bits 10...19 Tx audio gain
      | Bit 20 unused
      | Bit 21 AM_Mode
      | Bit 22 CW_nSSB
      | Bit 23 TX_Mon
      | Bit 24 LSB_USB
      | Bit 25 Tx_Rx
  Din : Inport
  Write : Inport  Port=2
  Down Sample : xbsIndex_r4/Down Sample  sample_ratio=1024  sample_phase="Last Value of Frame  (most efficient)"  en=off  latency=1  dbl_ovrd=off  block_type=dsamp
      settings: block_version=9.2.00
  RX Level : xbsIndex_r4/Slice  nbits=10  boolean_output=off  mode=Lower Bit Location + Width  bit1=-2  base1=MSB of Input  bit0=0  base0=LSB of Input  dbl_ovrd=off  block_type=slice
      settings: infoedit="Extracts a given range of bits from each input sample and presents it at the output.  The output type is ordinarily unsigned with binary point at zero, but can be Boolean when the slice is one bit wide.<P><P>Hardware notes: In hardware this block costs nothing."  block_version=9.2.00
  Register : xbsIndex_r4/Register  init=0  rst=off  en=on  dbl_ovrd=off  block_type=register
      settings: block_version=9.2.00
  Reinterpret : xbsIndex_r4/Reinterpret  force_arith_type=on  arith_type=Unsigned  force_bin_pt=on  bin_pt=10  block_type=reinterpret
      settings: infoedit="Changes signal type without altering the binary representation.   You can changed the signal between signed and unsigned, and relocate the binary point.<br><br>Hardware notes: In hardware this block costs nothing.<br><br>Example:  Suppose the input is 6 bits wide, signed, with 2 fractional bits, and the output is forced to unsigned with 0 fractional bits.  Then an input of -2.0 (1110.00 in binary 2's complement) becomes an output of 56 (111000 in binary)."  block_version=9.2.00
  Reinterpret1 : xbsIndex_r4/Reinterpret  force_arith_type=on  arith_type=Unsigned  force_bin_pt=on  bin_pt=10  block_type=reinterpret
      settings: infoedit="Changes signal type without altering the binary representation.   You can changed the signal between signed and unsigned, and relocate the binary point.<br><br>Hardware notes: In hardware this block costs nothing.<br><br>Example:  Suppose the input is 6 bits wide, signed, with 2 fractional bits, and the output is forced to unsigned with 0 fractional bits.  Then an input of -2.0 (1110.00 in binary 2's complement) becomes an output of 56 (111000 in binary)."  block_version=9.2.00
  Slice : xbsIndex_r4/Slice  nbits=1  boolean_output=on  mode=Upper Bit Location + Width  bit1=0  base1=MSB of Input  bit0=0  base0=LSB of Input  dbl_ovrd=off  block_type=slice
      settings: infoedit="Extracts a given range of bits from each input sample and presents it at the output.  The output type is ordinarily unsigned with binary point at zero, but can be Boolean when the slice is one bit wide.<P><P>Hardware notes: In hardware this block costs nothing."  block_version=9.2.00
  Slice1 : xbsIndex_r4/Slice  nbits=1  boolean_output=on  mode=Upper Bit Location + Width  bit1=-1  base1=MSB of Input  bit0=0  base0=LSB of Input  dbl_ovrd=off  block_type=slice
      settings: infoedit="Extracts a given range of bits from each input sample and presents it at the output.  The output type is ordinarily unsigned with binary point at zero, but can be Boolean when the slice is one bit wide.<P><P>Hardware notes: In hardware this block costs nothing."  block_version=9.2.00
  Slice2 : xbsIndex_r4/Slice  nbits=1  boolean_output=on  mode=Upper Bit Location + Width  bit1=-3  base1=MSB of Input  bit0=0  base0=LSB of Input  dbl_ovrd=off  block_type=slice
      settings: infoedit="Extracts a given range of bits from each input sample and presents it at the output.  The output type is ordinarily unsigned with binary point at zero, but can be Boolean when the slice is one bit wide.<P><P>Hardware notes: In hardware this block costs nothing."  block_version=9.2.00
  Slice3 : xbsIndex_r4/Slice  nbits=1  boolean_output=on  mode=Upper Bit Location + Width  bit1=-4  base1=MSB of Input  bit0=0  base0=LSB of Input  dbl_ovrd=off  block_type=slice
      settings: block_version=9.2.00
  Slice5 : xbsIndex_r4/Slice  nbits=1  boolean_output=on  mode=Upper Bit Location + Width  bit1=-2  base1=MSB of Input  bit0=0  base0=LSB of Input  dbl_ovrd=off  block_type=slice
      settings: infoedit="Extracts a given range of bits from each input sample and presents it at the output.  The output type is ordinarily unsigned with binary point at zero, but can be Boolean when the slice is one bit wide.<P><P>Hardware notes: In hardware this block costs nothing."  block_version=9.2.00
  TX Level : xbsIndex_r4/Slice  nbits=10  boolean_output=off  mode=Lower Bit Location + Width  bit1=-2  base1=MSB of Input  bit0=10  base0=LSB of Input  dbl_ovrd=off  block_type=slice
      settings: infoedit="Extracts a given range of bits from each input sample and presents it at the output.  The output type is ordinarily unsigned with binary point at zero, but can be Boolean when the slice is one bit wide.<P><P>Hardware notes: In hardware this block costs nothing."  block_version=9.2.00
  TX_Mon : Outport
  CW_nSSB : Outport  Port=2
  LSB_USB : Outport  Port=3
  AM_Mode : Outport  Port=4
  Tx_Rx_bit : Outport  Port=5
  Rx_Level : Outport  Port=6
  Tx_Level : Outport  Port=7
  wires:
  Down Sample/1 -> Slice1/1, Slice5/1, Slice2/1, Slice3/1, TX Level/1, RX Level/1, Slice/1
  Register/1 -> Down Sample/1
  Din/1 -> Register/1
  Slice/1 -> Tx_Rx_bit/1  "b25"
  Write/1 -> Register/2
  Slice1/1 -> LSB_USB/1  "b24"
  Slice5/1 -> TX_Mon/1  "b23"
  Slice2/1 -> CW_nSSB/1  "b22_CW_nSSB"
  RX Level/1 -> Reinterpret/1
  TX Level/1 -> Reinterpret1/1
  Reinterpret/1 -> Rx_Level/1
  Reinterpret1/1 -> Tx_Level/1  "X"
  Slice3/1 -> AM_Mode/1  "b21_AM"

== system Xcvr_SSB_AM_2p5/Audio_and_Mode_Control/Reg_B ==
  note: Reg_B
      | Bits 0..9 for SideTone level control
      | Bits 10..21 set TR Hang Delay
      | Bit 22 Two Tone Gen
      |
      | Bit 23 Post Rx CIC Gain_0
      | Bit 24 Post Rx CIC Gain_1
      |            Bit 1  Bit 0   Gain in dB
      |               0      0         0
      |               0      1         6
      |               1      0        12
      |               1      1        18
  Din : Inport
  Write : Inport  Port=2
  Down Sample1 : xbsIndex_r4/Down Sample  sample_ratio=1024  sample_phase="Last Value of Frame  (most efficient)"  en=off  latency=1  dbl_ovrd=off  block_type=dsamp
      settings: block_version=9.2.00
  Post_CIC_Bit_23 : xbsIndex_r4/Slice  nbits=1  boolean_output=on  mode=Upper Bit Location + Width  bit1=-2  base1=MSB of Input  bit0=0  base0=LSB of Input  dbl_ovrd=off  block_type=slice
      settings: block_version=9.2.00
  Post_DA_Bit _24 : xbsIndex_r4/Slice  nbits=1  boolean_output=on  mode=Upper Bit Location + Width  bit1=-1  base1=MSB of Input  bit0=0  base0=LSB of Input  dbl_ovrd=off  block_type=slice
      settings: block_version=9.2.00
  Register1 : xbsIndex_r4/Register  init=0  rst=off  en=on  dbl_ovrd=off  block_type=register
      settings: block_version=9.2.00
  Reinterpret1 : xbsIndex_r4/Reinterpret  force_arith_type=on  arith_type=Unsigned  force_bin_pt=on  bin_pt=10  block_type=reinterpret
      settings: infoedit="Changes signal type without altering the binary representation.   You can changed the signal between signed and unsigned, and relocate the binary point.<br><br>Hardware notes: In hardware this block costs nothing.<br><br>Example:  Suppose the input is 6 bits wide, signed, with 2 fractional bits, and the output is forced to unsigned with 0 fractional bits.  Then an input of -2.0 (1110.00 in binary 2's complement) becomes an output of 56 (111000 in binary)."  block_version=9.2.00
  Reinterpret2 : xbsIndex_r4/Reinterpret  force_arith_type=on  arith_type=Unsigned  force_bin_pt=on  bin_pt=0  block_type=reinterpret
      settings: infoedit="Changes signal type without altering the binary representation.   You can changed the signal between signed and unsigned, and relocate the binary point.<P><P>Hardware notes: In hardware this block costs nothing.<P><P>Example:  Suppose the input is 6 bits wide, signed, with 2 fractional bits, and the output is forced to unsigned with 0 fractional bits.  Then an input of -2.0 (1110.00 in binary 2's complement) becomes an output of 56 (111000 in binary)."  block_version=9.2.00
  SideTone Level1 : xbsIndex_r4/Slice  nbits=10  boolean_output=off  mode=Lower Bit Location + Width  bit1=-2  base1=MSB of Input  bit0=0  base0=LSB of Input  dbl_ovrd=off  block_type=slice
      settings: block_version=9.2.00
  TRD : xbsIndex_r4/Slice  nbits=12  boolean_output=off  mode=Lower Bit Location + Width  bit1=-2  base1=MSB of Input  bit0=10  base0=LSB of Input  dbl_ovrd=off  block_type=slice
      settings: block_version=9.2.00
  Two_Tone_Bit_22 : xbsIndex_r4/Slice  nbits=1  boolean_output=on  mode=Upper Bit Location + Width  bit1=-3  base1=MSB of Input  bit0=0  base0=LSB of Input  dbl_ovrd=off  block_type=slice
      settings: block_version=9.2.00
  Side_Tone_Level : Outport
  Two_Tone : Outport  Port=2
  Post_CIC_Gain_0 : Outport  Port=3
  Post_CIC_Gain_1 : Outport  Port=4
  TR Delay : Outport  Port=5
  wires:
  Down Sample1/1 -> SideTone Level1/1, TRD/1, Two_Tone_Bit_22/1, Post_CIC_Bit_23/1, Post_DA_Bit _24/1
  TRD/1 -> Reinterpret2/1
  SideTone Level1/1 -> Reinterpret1/1
  Reinterpret1/1 -> Side_Tone_Level/1
  Reinterpret2/1 -> TR Delay/1
  Two_Tone_Bit_22/1 -> Two_Tone/1
  Register1/1 -> Down Sample1/1
  Din/1 -> Register1/1
  Write/1 -> Register1/2
  Post_CIC_Bit_23/1 -> Post_CIC_Gain_0/1
  Post_DA_Bit _24/1 -> Post_CIC_Gain_1/1

== system Xcvr_SSB_AM_2p5/Audio_and_Mode_Control/T_R_Delay ==
  note: ^ Inserted serial delay here
      | to delay Tx (to help preserve
      | length of iniial CW character, which
      | normally is clipped by about 13 ms).
  Tx_Rx_bit : Inport  OutDataType=sfix(16)  OutScaling=2^0
  Delay : Inport  Port=2  OutDataType=sfix(16)  OutScaling=2^0
  Constant1 : xbsIndex_r4/Constant  arith_type=Unsigned  const=40  n_bits=6  bin_pt=0  explicit_period=off  period=1  equ=P=C  opselect=C  inp2=PCIN>>17  opr=+  inp1=P  carry=CIN  dbl_ovrd=off  block_type=constant
      settings: block_version=12.1
  Constant2 : xbsIndex_r4/Constant  arith_type=Unsigned  const=0  n_bits=13  bin_pt=0  explicit_period=off  period=1  equ=P=C  opselect=C  inp2=PCIN>>17  opr=+  inp1=P  carry=CIN  dbl_ovrd=off  block_type=constant
      settings: block_version=12.1
  Counter : xbsIndex_r4/Counter  cnt_type=Free Running  cnt_to=0  operation=Down  start_count=0  cnt_by_val=1  arith_type=Unsigned  n_bits=12  bin_pt=0  load_pin=on  rst=off  en=on  explicit_period=off  period=1/Faudio  dbl_ovrd=off  use_behavioral_HDL=off  implementation=Fabric  block_type=counter
      settings: block_version=12.1
  Counter1 : xbsIndex_r4/Counter  cnt_type=Free Running  cnt_to=47  operation=Up  start_count=0  cnt_by_val=1  arith_type=Unsigned  n_bits=6  bin_pt=0  load_pin=off  rst=on  en=on  explicit_period=off  period=1  dbl_ovrd=off  use_behavioral_HDL=off  implementation=Fabric  block_type=counter
      settings: block_version=12.1
  Delay1 : xbsIndex_r4/Delay  en=off  latency=160  dbl_ovrd=off  reg_retiming=off  block_type=delay
      settings: block_version=9.2.00
  Delay2 : xbsIndex_r4/Delay  en=off  latency=1  dbl_ovrd=off  reg_retiming=off  block_type=delay
      settings: block_version=9.2.00
  Delay5 : xbsIndex_r4/Delay  en=off  latency=1  dbl_ovrd=off  reg_retiming=off  block_type=delay
      settings: block_version=9.2.00
  Inverter{1..4} (4 alike) : xbsIndex_r4/Inverter  en=off  latency=0  dbl_ovrd=off  block_type=inv
      settings: block_version=9.2.00
  Logical1 : xbsIndex_r4/Logical  logical_function=AND  inputs=2  en=off  latency=0  precision=Full  arith_type=Unsigned  n_bits=16  bin_pt=0  align_bp=on  dbl_ovrd=off  block_type=logical
      settings: block_version=12.1
  Logical2 : xbsIndex_r4/Logical  logical_function=AND  inputs=2  en=off  latency=0  precision=Full  arith_type=Unsigned  n_bits=16  bin_pt=0  align_bp=on  dbl_ovrd=off  block_type=logical
      settings: block_version=12.1
  Logical3 : xbsIndex_r4/Logical  logical_function=OR  inputs=2  en=off  latency=0  precision=Full  arith_type=Unsigned  n_bits=16  bin_pt=0  align_bp=on  dbl_ovrd=off  block_type=logical
      settings: block_version=12.1
  Logical4 : xbsIndex_r4/Logical  logical_function=OR  inputs=3  en=off  latency=0  precision=Full  arith_type=Unsigned  n_bits=16  bin_pt=0  align_bp=on  dbl_ovrd=off  block_type=logical
      settings: block_version=12.1
  Relational : xbsIndex_r4/Relational  mode=a=b  en=off  latency=0  dbl_ovrd=off  block_type=relational
      settings: block_version=9.2.00
  Relational1 : xbsIndex_r4/Relational  mode=a=b  en=off  latency=0  dbl_ovrd=off  block_type=relational
      settings: block_version=9.2.00
  Tx_Rx_D40 : Outport
  Tx_RX : Outport  Port=2
  Tx_RX_Delayed : Outport  Port=3
  wires:
  Tx_Rx_bit/1 -> Delay2/1, Inverter2/1, Logical4/1
  Delay2/1 -> Logical2/2, Logical4/2, Delay1/1
  Constant2/1 -> Relational/2
  Counter/1 -> Relational/1
  Relational/1 -> Inverter1/1
  Inverter1/1 -> Logical3/2, Logical4/3
  Logical3/1 -> Counter/3
  Delay/1 -> Counter/2
  Inverter2/1 -> Logical2/1
  Logical2/1 -> Counter/1, Logical3/1
  Logical4/1 -> Delay5/1
  Delay5/1 -> Tx_RX_Delayed/1, Logical1/1, Inverter3/1
  Counter1/1 -> Relational1/1
  Relational1/1 -> Logical1/2, Inverter4/1
  Inverter3/1 -> Counter1/1
  Constant1/1 -> Relational1/2
  Inverter4/1 -> Counter1/2
  Logical1/1 -> Tx_Rx_D40/1
  Delay1/1 -> Tx_RX/1
